simulink model "motor_real"  (R2023b)
settings: Solver=FixedStepAuto  StartTime=0.0  StopTime=5  RelTol=1e-3  EnableMultiTasking=on
libraries: mbedblockslib x6, simulink x1
settings Model: ExtModeTrigDuration=10  Creator=miqui  LastModifiedBy=miqui
settings OptimizationCC: EnhancedBackFolding=on  PassReuseOutputArgsAs=Individual arguments  ZeroExternalMemoryAtStartup=off  ZeroInternalMemoryAtStartup=off  MaxStackSize=64  OptimizeBlockOrder=speed  DifferentSizesBufferReuse=on  OptimizationCustomize=off  EfficientTunableParamExpr=on
settings DebuggingCC: ParameterTunabilityLossMsg=error
settings HardwareCC: ProdBitPerPointer=32  ProdBitPerSizeT=32  ProdBitPerPtrDiffT=32  ProdLargestAtomicInteger=Long  ProdLargestAtomicFloat=Double  ProdWordSize=32  ProdLongLongMode=on  ProdHWDeviceType=ARM Compatible->ARM Cortex  UseEmbeddedCoderFeatures=off
settings SFSimCC: MATLABDynamicMemAlloc=off
settings RTWCC: Description=Embedded Coder  SystemTargetFile=ert.tlc  HardwareBoard=STM32 Nucleo F411RE  TemplateMakefile=ert_default_tmf  Toolchain=GNU Tools for ARM Embedded Processors
settings CodeAppCC: ForceParamTrailComments=on  IgnoreCustomStorageClasses=off  OperatorAnnotations=on  SimulinkDataObjDesc=on  SFDataObjDesc=on  InsertBlockDesc=on
settings ERTTargetCC: SupportNonInlinedSFcns=on  ExtModeTransport=3  ExtModeStaticAlloc=on  ExtModeStaticAllocSize=2000  ExtModeMexFile=ext_xcp  ExtModeIntrfLevel=Level2 - Open

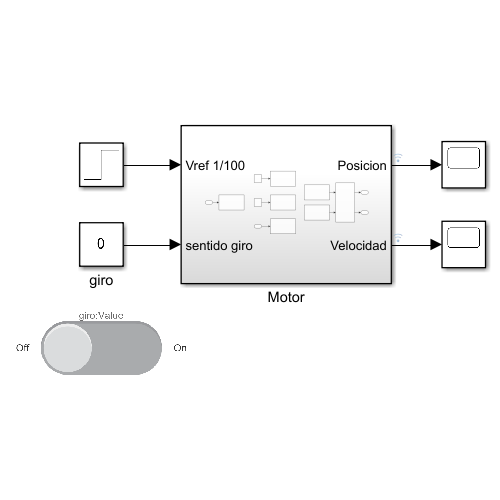
[thumbnail: Simulink's stored preview of the top-level diagram]
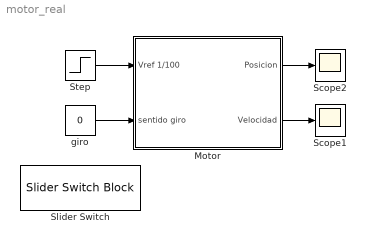
== system motor_real ==
  Motor : Subsystem
  Scope1 : Scope
  Scope2 : Scope
  Slider Switch : SliderSwitchBlock
      settings: Values={{'Off', 'On'}, [0 1]}
  Step : Step  After=0  SampleTime=0.1
  giro : Constant  Value=0
  wires:
  Step/1 -> Motor/1(Vref 1/100)
  giro/1 -> Motor/2(sentido giro)
  Motor/1(Posicion) -> Scope2/1
  Motor/2(Velocidad) -> Scope1/1

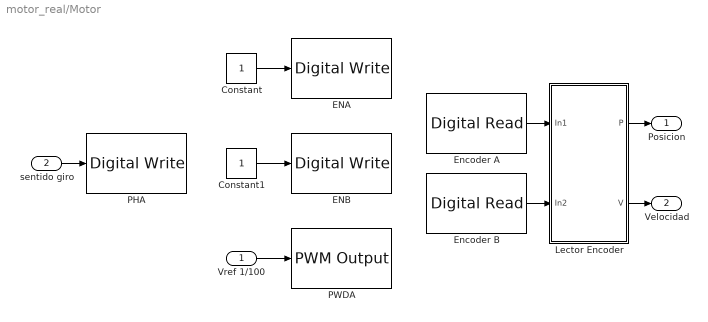
== system motor_real/Motor ==
  Vref 1/100 : Inport
  sentido giro : Inport  Port=2
  Constant : Constant
  Constant1 : Constant
  ENA : mbedblockslib/Digital Write  Pin=D2  Direction=output
      settings: LibrarySourceBlock=stmnucleorootlib/Common/Digital Write
  ENB : mbedblockslib/Digital Write  Pin=D11  Direction=output
      settings: LibrarySourceBlock=stmnucleorootlib/Common/Digital Write
  Encoder A : mbedblockslib/Digital Read  Pin=A1  Direction=input  SampleTime=0.0001
      settings: LibrarySourceBlock=stmnucleorootlib/Common/Digital Read
  Encoder B : mbedblockslib/Digital Read  Pin=A0  Direction=input  SampleTime=0.0001
      settings: LibrarySourceBlock=stmnucleorootlib/Common/Digital Read
  Lector Encoder : Subsystem
  PHA : mbedblockslib/Digital Write  Pin=D3  Direction=output
      settings: LibrarySourceBlock=stmnucleorootlib/Common/Digital Write
  PWDA : mbedblockslib/PWM Output  Pin=D5  EnableInputFrequency=off  InitialFrequency=5000  InitialDutyCycle=0  NotificationType=None
      settings: LibrarySourceBlock=stmnucleorootlib/Common/PWM Output
  Posicion : Outport
  Velocidad : Outport  Port=2
  wires:
  sentido giro/1 -> PHA/1
  Constant/1 -> ENA/1
  Constant1/1 -> ENB/1
  Vref 1/100/1 -> PWDA/1
  Encoder A/1 -> Lector Encoder/1(In1)
  Encoder B/1 -> Lector Encoder/2(In2)
  Lector Encoder/2(V) -> Velocidad/1
  Lector Encoder/1(P) -> Posicion/1

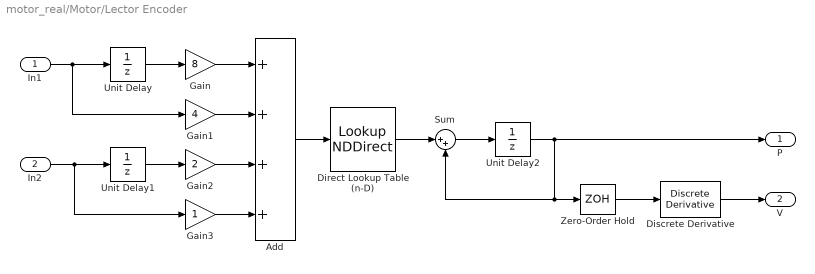
== system motor_real/Motor/Lector Encoder ==
  In1 : Inport
  In2 : Inport  Port=2
  Add : Sum  Inputs=++++  OutDataTypeStr=double
  Direct Lookup Table (n-D) : LookupNDDirect  NumberOfTableDimensions=1  Table=[0,-1,1,0,1,0,0,-1,-1,0,0,1,0,1,-1,0]
  Discrete Derivative : simulink/Discrete/Discrete Derivative  gainval=1.0  ICPrevScaledInput=0.0  OutMin=[]  OutMax=[]  OutDataType=fixdt(1, 16)  OutScaling=2^-10  DoSatur=off
  Gain : Gain  Gain=8
  Gain1 : Gain  Gain=4
  Gain2 : Gain  Gain=2
  Gain3 : Gain
  Sum : Sum  Inputs=|++
  Unit Delay : UnitDelay  SampleTime=-1  HasFrameUpgradeWarning=on
  Unit Delay1 : UnitDelay  SampleTime=-1  HasFrameUpgradeWarning=on
  Unit Delay2 : UnitDelay  SampleTime=-1  HasFrameUpgradeWarning=on
  Zero-Order Hold : ZeroOrderHold  SampleTime=0.01
  P : Outport
  V : Outport  Port=2
  wires:
  In1/1 -> Gain1/1, Unit Delay/1
  In2/1 -> Gain3/1, Unit Delay1/1
  Unit Delay/1 -> Gain/1
  Unit Delay1/1 -> Gain2/1
  Gain/1 -> Add/1
  Gain1/1 -> Add/2
  Gain2/1 -> Add/3
  Gain3/1 -> Add/4
  Add/1 -> Direct Lookup Table (n-D)/1
  Direct Lookup Table (n-D)/1 -> Sum/1
  Sum/1 -> Unit Delay2/1
  Unit Delay2/1 -> Zero-Order Hold/1, Sum/2, P/1
  Zero-Order Hold/1 -> Discrete Derivative/1
  Discrete Derivative/1 -> V/1
